simulink model "bai411"  (R2022b)
settings: Solver=VariableStepAuto  StartTime=0.0  StopTime=10.0  RelTol=1e-3
undefined symbols (not defined in the file or in its folder): k, s
settings Model: Creator=admin  LastModifiedBy=admin

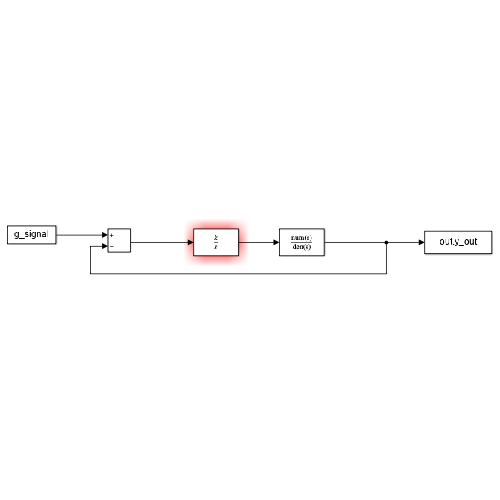
[thumbnail: Simulink's stored preview of the top-level diagram]
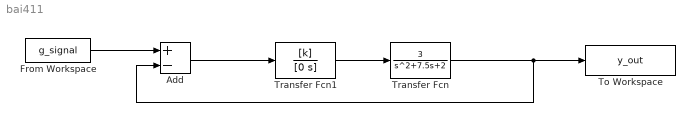
== system bai411 ==
  Add : Sum  Inputs=+-
  From Workspace : FromWorkspace  VariableName=g_signal
  To Workspace : ToWorkspace  VariableName=y_out  SaveFormat=Structure With Time  SampleTime=-1
  Transfer Fcn : TransferFcn  Numerator=[3]  Denominator=[1 7.5 2]
  Transfer Fcn1 : TransferFcn  Numerator=[k]  Denominator=[0 s]
  wires:
  Transfer Fcn/1 -> To Workspace/1, Add/2
  From Workspace/1 -> Add/1
  Transfer Fcn1/1 -> Transfer Fcn/1
  Add/1 -> Transfer Fcn1/1
